simulink model "untitled"  (R2017b)
settings: Solver=VariableStepAuto  StartTime=0.0  StopTime=10  RelTol=1e-3
undefined symbols (not defined in the file): a10, a20, aPrim10, aPrim20, L
settings Model: Creator=krzyl  LastModifiedBy=krzyl

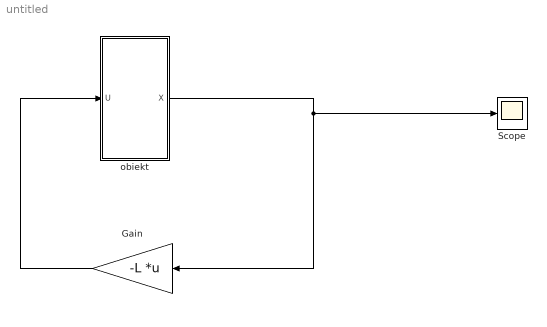
== system untitled ==
  Gain : Gain  Gain=-L  Multiplication=Matrix(K*u)
  Scope : Scope
  "obiekt " : Subsystem
  wires:
  "obiekt "/1(X) -> Scope/1, Gain/1
  Gain/1 -> "obiekt "/1(U)

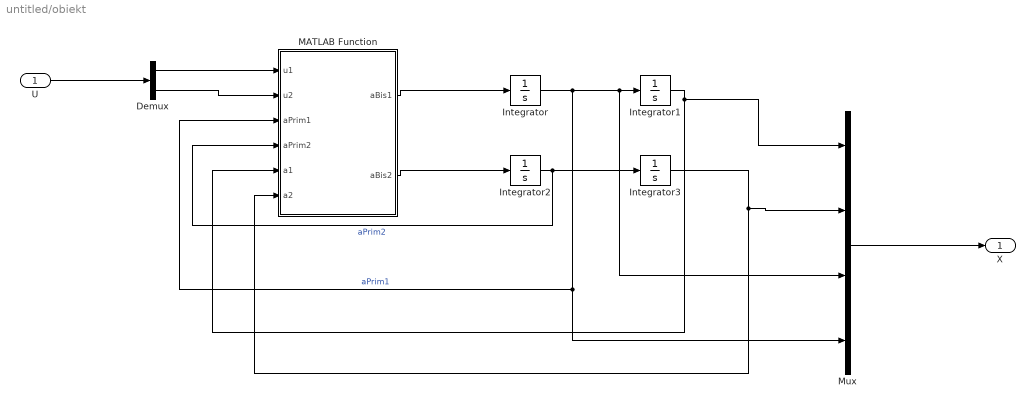
== system untitled/obiekt  ==
  U : Inport
  Demux : Demux  Outputs=2
  Integrator : Integrator  InitialCondition=aPrim10
  Integrator1 : Integrator  InitialCondition=a10
  Integrator2 : Integrator  InitialCondition=aPrim20
  Integrator3 : Integrator  InitialCondition=a20-0.001
  MATLAB Function : MATLAB Function  TreatAsAtomicUnit=on
  Mux : Mux
  X : Outport
  wires:
  MATLAB Function/2(aBis2) -> Integrator2/1
  Integrator2/1 -> Integrator3/1, MATLAB Function/4(aPrim2)  "aPrim2"
  Integrator/1 -> Mux/4, MATLAB Function/3(aPrim1), Mux/3, Integrator1/1  "aPrim1"
  MATLAB Function/1(aBis1) -> Integrator/1
  Mux/1 -> X/1
  Integrator3/1 -> Mux/2, MATLAB Function/6(a2)
  Integrator1/1 -> Mux/1, MATLAB Function/5(a1)
  U/1 -> Demux/1
  Demux/1 -> MATLAB Function/1(u1)
  Demux/2 -> MATLAB Function/2(u2)

== matlab function untitled/obiekt /MATLAB Function ==
  data: u1 input; u2 input; aBis1 output; aPrim1 input; aPrim2 input; a1 input; a2 input; aBis2 output
function [aBis1, aBis2] = fcn(u1, u2, aPrim1, aPrim2, a1, a2)

    m1 = 2; m2 = 1; l1 = 1.5; l2 = 1; lc1 = l1/2; lc2 = l2/2; J1 = m1*lc1^2; J2 = m2*lc2^2; g = 9.81;
    H11 = m1*lc1^2 + J1 + m2*(l1^2 + lc2^2 + 2*l1*l2*cos(a2)) + J2;
    H12  = m2*l1*lc2*cos(a2) + m2*lc2^2 + J2;
    H21 = H12;
    H22 = m2*lc2^2 + J2;
    h = m2*l1*lc2*sin(a2);
    g1 = m1*lc1*g*cos(a1) + m2*g*(lc2*cos(a1+a2)+l1*cos(a1));
    g2 = m2*lc2*g*cos(a1+a2);
    H = [H11 H12; H21 H22];
    H2 = inv(H);

    J = [-h*aPrim2, -h*aPrim1-h*aPrim2; h*aPrim1,0];
    M = [g1;g2];
    U = [u1;u2];
    %rozwikłanie 
    Roz = -1*H2*J*[aPrim1; aPrim2] -1*H2*M + H2*U; 
    aBis = Roz;% simplify(Roz);
   
    aBis1 = aBis(1);
    aBis2 = aBis(2);
end
